simulink model "PROJECTQ5"  (R2022a)
settings: Solver=VariableStepAuto  StartTime=0.0  StopTime=10.0  RelTol=1e-3
settings Model: Creator=1234567890  LastModifiedBy=1234567890

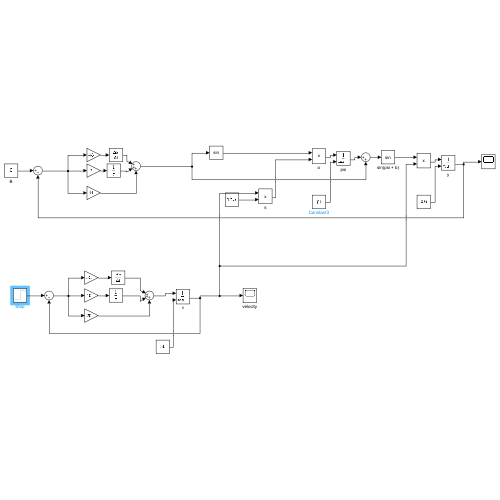
[thumbnail: Simulink's stored preview of the top-level diagram]
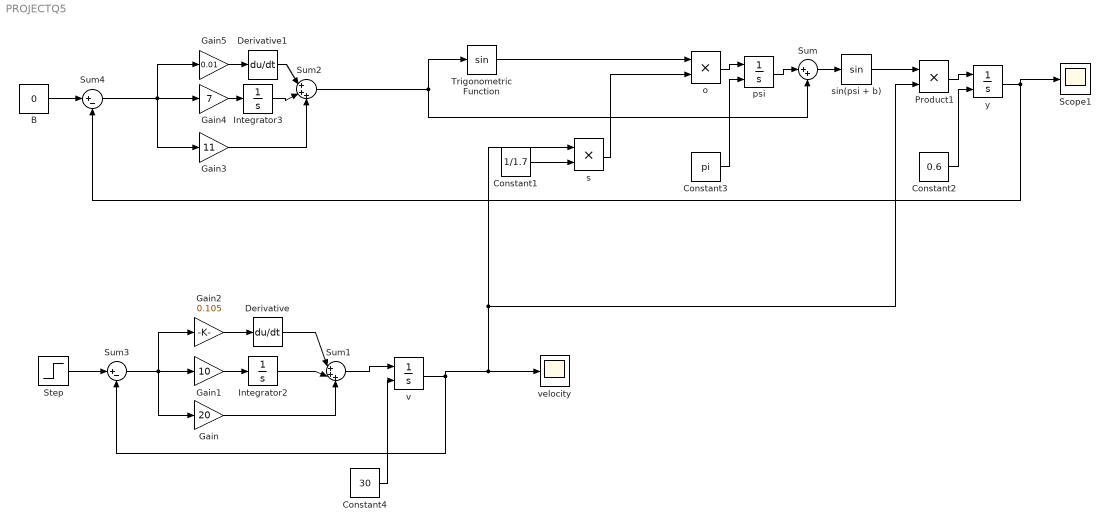
== system PROJECTQ5 ==
  B : Constant  Value=0
  Constant1 : Constant  Value=1/1.7
  Constant2 : Constant  Value=0.6
  Constant3 : Constant  Value=pi
  Constant4 : Constant  Value=30
  Derivative : Derivative
  Derivative1 : Derivative
  Gain : Gain  Gain=20
  Gain1 : Gain  Gain=10
  Gain2 : Gain  Gain=0.105
  Gain3 : Gain  Gain=11
  Gain4 : Gain  Gain=7
  Gain5 : Gain  Gain=0.01
  Integrator2 : Integrator
  Integrator3 : Integrator
  Product1 : Product
  Scope1 : Scope
  Step : Step  Time=0  Before=15.65  After=15.65  SampleTime=0
  Sum : Sum  Inputs=|++
  Sum1 : Sum  Inputs=|+++
  Sum2 : Sum  Inputs=|+++
  Sum3 : Sum  Inputs=|+-
  Sum4 : Sum  Inputs=|+-
  Trigonometric Function : Trigonometry
  o : Product
  psi : Integrator  InitialConditionSource=external
  s : Product
  sin(psi + b) : Trigonometry
  v : Integrator  InitialConditionSource=external
  velocity : Scope
  y : Integrator  InitialConditionSource=external
  wires:
  v/1 -> velocity/1, Product1/2, s/1, Sum3/2
  Trigonometric Function/1 -> o/1
  o/1 -> psi/1
  psi/1 -> Sum/1
  Sum/1 -> sin(psi + b)/1
  sin(psi + b)/1 -> Product1/1
  Product1/1 -> y/1
  y/1 -> Scope1/1, Sum4/2
  Gain2/1 -> Derivative/1
  Sum1/1 -> v/1
  Derivative/1 -> Sum1/1
  Gain1/1 -> Integrator2/1
  Integrator2/1 -> Sum1/2
  Gain/1 -> Sum1/3
  Integrator3/1 -> Sum2/2
  Sum2/1 -> Sum/2, Trigonometric Function/1
  Gain4/1 -> Integrator3/1
  Gain3/1 -> Sum2/3
  Gain5/1 -> Derivative1/1
  Derivative1/1 -> Sum2/1
  Constant1/1 -> s/2
  s/1 -> o/2
  Step/1 -> Sum3/1
  Sum3/1 -> Gain/1, Gain2/1, Gain1/1
  B/1 -> Sum4/1
  Sum4/1 -> Gain4/1, Gain3/1, Gain5/1
  Constant2/1 -> y/2
  Constant3/1 -> psi/2
  Constant4/1 -> v/2
